simulink model "PID_ctrl"  (R2022b)
settings: Solver=FixedStepDiscrete  StartTime=0.0  StopTime=100.0  FixedStep=0.01  RelTol=1e-3
settings Model: Creator=yasso  LastModifiedBy=yasso
settings OptimizationCC: DefaultParameterBehavior=Inlined  UseDivisionForNetSlopeComputation=on  GainParamInheritBuiltInType=on  UseFloatMulNetSlope=on  InlineInvariantSignals=on  PassReuseOutputArgsAs=Individual arguments  ZeroExternalMemoryAtStartup=off  ZeroInternalMemoryAtStartup=off  NoFixptDivByZeroProtection=on  EfficientFloat2IntCast=on  LifeSpan=1  OptimizeBlockOrder=speed  DifferentSizesBufferReuse=on  EfficientTunableParamExpr=on
settings DebuggingCC: ParameterTunabilityLossMsg=error
settings HardwareCC: ProdLongLongMode=on
settings SFSimCC: MATLABDynamicMemAlloc=off
settings RTWCC: Description=Embedded Coder  SystemTargetFile=ert.tlc  TemplateMakefile=ert_default_tmf  CreateSILPILBlock=SIL
settings CodeAppCC: ForceParamTrailComments=on  IgnoreCustomStorageClasses=off  OperatorAnnotations=on  SimulinkDataObjDesc=on  SFDataObjDesc=on  CustomSymbolStrGlobalVar=rt$N$M  CustomSymbolStrType=$N$M  CustomSymbolStrFcn=$N$M$F  CustomSymbolStrMacro=$N$M  InsertBlockDesc=on
settings ERTTargetCC: TargetLangStandard=C99 (ISO)  GenerateSampleERTMain=on  IncludeMdlTerminateFcn=off  CombineSignalStateStructs=on  SuppressErrorStatus=on  SupportAbsoluteTime=off  SupportComplex=off  InlinedParameterPlacement=NonHierarchical  ERTCustomFileTemplate=example_file_process.tlc  ERTFilePackagingFormat=CompactWithDataFile

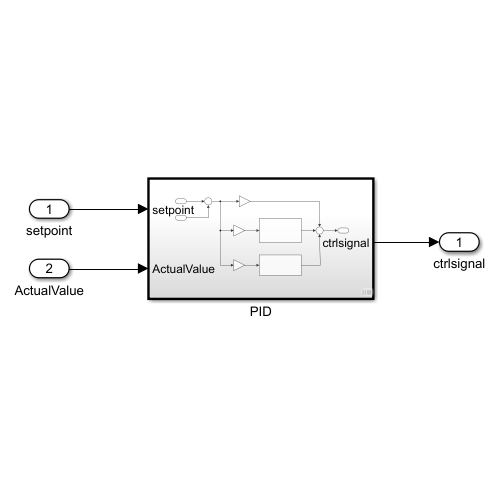
[thumbnail: Simulink's stored preview of the top-level diagram]
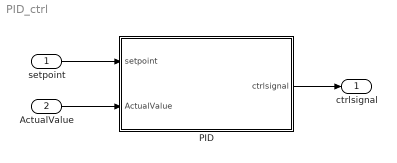
== system PID_ctrl ==
  setpoint : Inport
  ActualValue : Inport  Port=2
  PID : Subsystem  TreatAsAtomicUnit=on
  ctrlsignal : Outport
  wires:
  setpoint/1 -> PID/1(setpoint)
  PID/1(ctrlsignal) -> ctrlsignal/1
  ActualValue/1 -> PID/2(ActualValue)

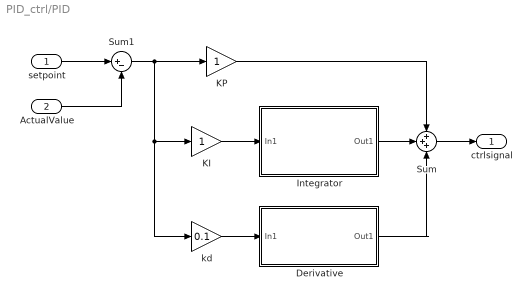
== system PID_ctrl/PID ==
  setpoint : Inport
  ActualValue : Inport  Port=2
  Derivative : Subsystem
  Integrator : Subsystem
  KI : Gain
  KP : Gain
  Sum : Sum  Inputs=+++
  Sum1 : Sum  Inputs=|+-
  kd : Gain  Gain=0.1
  ctrlsignal : Outport
  wires:
  Sum1/1 -> KI/1, kd/1, KP/1
  setpoint/1 -> Sum1/1
  ActualValue/1 -> Sum1/2
  KI/1 -> Integrator/1(In1)
  Derivative/1(Out1) -> Sum/3
  kd/1 -> Derivative/1(In1)
  KP/1 -> Sum/1
  Integrator/1(Out1) -> Sum/2
  Sum/1 -> ctrlsignal/1

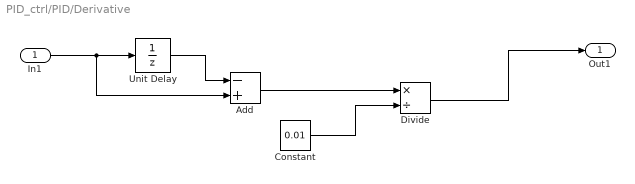
== system PID_ctrl/PID/Derivative ==
  In1 : Inport
  Add : Sum  Inputs=-+
  Constant : Constant  Value=0.01
  Divide : Product  Inputs=*/
  Unit Delay : UnitDelay  SampleTime=-1  HasFrameUpgradeWarning=on
  Out1 : Outport
  wires:
  In1/1 -> Add/2, Unit Delay/1
  Unit Delay/1 -> Add/1
  Add/1 -> Divide/1
  Constant/1 -> Divide/2
  Divide/1 -> Out1/1

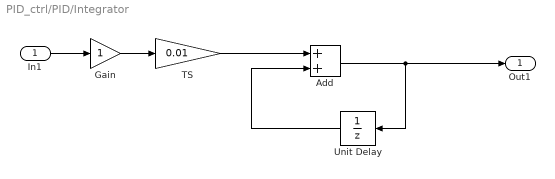
== system PID_ctrl/PID/Integrator ==
  In1 : Inport
  Add : Sum
  Gain : Gain
  TS : Gain  Gain=0.01
  Unit Delay : UnitDelay  SampleTime=-1  HasFrameUpgradeWarning=on
  Out1 : Outport
  wires:
  Add/1 -> Unit Delay/1, Out1/1
  Unit Delay/1 -> Add/2
  In1/1 -> Gain/1
  TS/1 -> Add/1
  Gain/1 -> TS/1
